simulink model "Controller"  (R2023b)
settings: Solver=VariableStepAuto  StartTime=0.0  StopTime=10.0  RelTol=1e-3
undefined symbols (not defined in the file): Kd, Ki, Kp, Ts
settings Model: Creator=siva kumar  LastModifiedBy=siva kumar
settings DataIOCC: SaveOutput=off  SaveTime=off

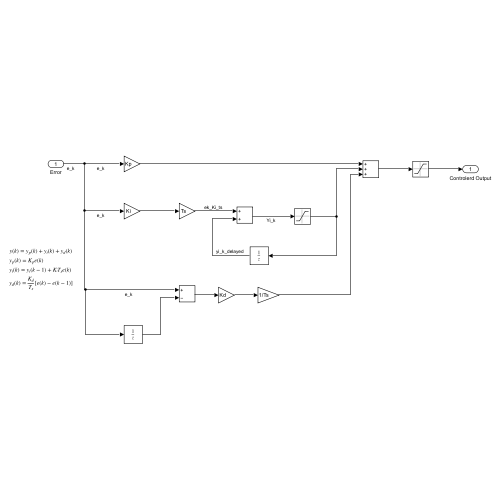
[thumbnail: Simulink's stored preview of the top-level diagram]
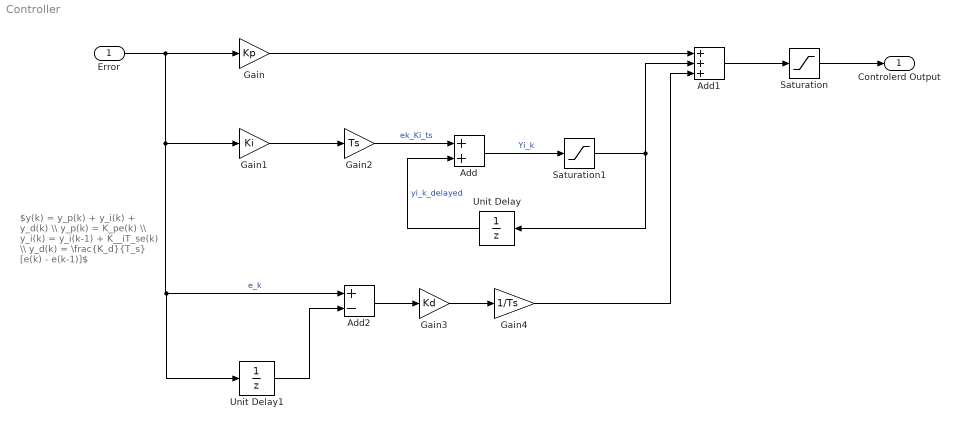
== system Controller ==
  note: $y(k) = y_p(k) + y_i(k) + y_d(k) \\ y_p(k) = K_pe(k) \\ y_i(k) = y_i(k-1) + K__iT_se(k) \\ y_d(k) = \frac{K_d}{T_s} [e(k) - e(k-1)]$
  Error : Inport  OutDataTypeStr=double  PortDimensions=1  SampleTime=[0,1]
  Add : Sum
  Add1 : Sum  Inputs=+++
  Add2 : Sum  Inputs=+-
  Gain : Gain  Gain=Kp
  Gain1 : Gain  Gain=Ki
  Gain2 : Gain  Gain=Ts
  Gain3 : Gain  Gain=Kd
  Gain4 : Gain  Gain=1/Ts
  Saturation : Saturate  UpperLimit=100  LowerLimit=-100
  Saturation1 : Saturate  UpperLimit=10  LowerLimit=-10
  Unit Delay : UnitDelay  SampleTime=-1  HasFrameUpgradeWarning=on
  Unit Delay1 : UnitDelay  SampleTime=-1  HasFrameUpgradeWarning=on
  Controlerd Output : Outport  OutDataTypeStr=double  PortDimensions=1  SampleTime=[0,1]
  wires:
  Error/1 -> Unit Delay1/1, Add2/1, Gain1/1, Gain/1  "e_k"
  Saturation/1 -> Controlerd Output/1
  Gain1/1 -> Gain2/1
  Gain2/1 -> Add/1  "ek_Ki_ts"
  Unit Delay/1 -> Add/2  "yi_k_delayed"
  Add/1 -> Saturation1/1  "Yi_k"
  Gain/1 -> Add1/1
  Add1/1 -> Saturation/1
  Unit Delay1/1 -> Add2/2
  Add2/1 -> Gain3/1
  Gain3/1 -> Gain4/1
  Gain4/1 -> Add1/3
  Saturation1/1 -> Add1/2, Unit Delay/1
